simulink model "gm_sampleModel1821_4_sub_sub_sub"  (R2023a)
settings: Solver=VariableStepAuto  StartTime=0.0  StopTime=10.0  RelTol=1e-3
libraries: hdlsllib x3
settings Model: Creator=user1  LastModifiedBy=user1
settings OptimizationCC: BlockReduction=off  ConditionallyExecuteInputs=off
settings DebuggingCC: InheritedTsInSrcMsg=none

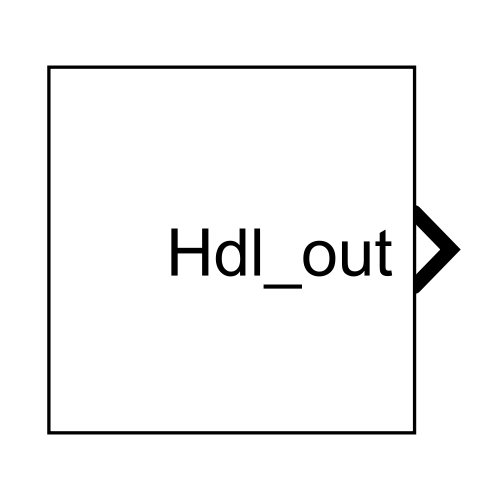
[thumbnail: Simulink's stored preview of the top-level diagram]
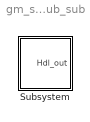
== system gm_sampleModel1821_4_sub_sub_sub ==
  Subsystem : Subsystem

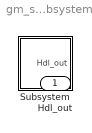
== system gm_sampleModel1821_4_sub_sub_sub/Subsystem ==
  Subsystem : Subsystem
  Hdl_out : Outport  OutDataTypeStr=uint8

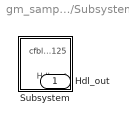
== system gm_sampleModel1821_4_sub_sub_sub/Subsystem/Subsystem ==
  Subsystem : Subsystem
  Hdl_out : Outport  OutDataTypeStr=uint8

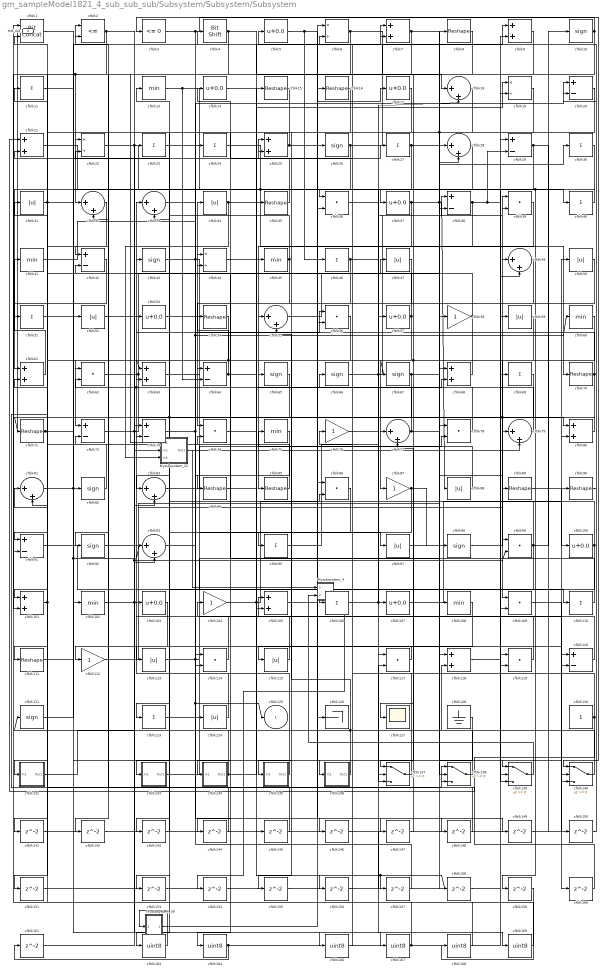
== system gm_sampleModel1821_4_sub_sub_sub/Subsystem/Subsystem/Subsystem ==
  Mysubsystem_22 : Subsystem  TreatAsAtomicUnit=on  RTWFcnName=Mysubsystem_22
      settings: RTWFcnNameOpts=User specified  RTWFileNameOpts=Use function name
  Mysubsystem_39 : Subsystem  TreatAsAtomicUnit=on  RTWFcnName=Mysubsystem_39
      settings: RTWFcnNameOpts=User specified  RTWFileNameOpts=Use function name
  Mysubsystem_4 : Subsystem  TreatAsAtomicUnit=on  RTWFcnName=Mysubsystem_4
      settings: RTWFcnNameOpts=User specified  RTWFileNameOpts=Use function name
  cfblk1 : hdlsllib/Logic and Bit Operations/Bit Concat  numInputs=2
  cfblk{10,26,43,65..67,82,92,98,121} (10 alike) : Signum
  cfblk{5,14,17,37,53,57,100,103,107} (9 alike) : Bias  Bias=0.0  SaturateOnIntegerOverflow=off
  cfblk{7,9,21,25,61,63,68,80,101,105,118} (11 alike) : Sum  OutDataTypeStr=uint8
  cfblk{13,41,45,60,75,102,108} (7 alike) : MinMax  OutDataTypeStr=uint8
  cfblk{58,76,87,104,112} (5 alike) : Gain  OutDataTypeStr=uint8
  cfblk{11,23..24,27,30,40,46,51,69,95,106,110,123} (13 alike) : Sum  Inputs=+  OutDataTypeStr=uint8
  cfblk{36,39,56,62,74,78,86,99,109,114,117,119} (12 alike) : DotProduct  OutDataTypeStr=uint8
  cfblk{8,15..16,35,54,70..71,84..85,89..90,111} (12 alike) : Reshape
  cfblk{31,34,47,50,52,59,88,97,113,115,124} (11 alike) : Abs  OutDataTypeStr=uint8  SaturateOnIntegerOverflow=off
  cfblk{20,29,38,42,64,72..73,91,120} (9 alike) : Sum  Inputs=+-  OutDataTypeStr=uint8
  cfblk126 : Terminator
  cfblk127 : Scope
  cfblk128 : Ground
  cfblk130 : Constant  OutDataTypeStr=uint8  SampleTime=-1
  cfblk131 : Subsystem
      settings: LibrarySourceBlock=|
      | hdlsllib/Ports &
      | Subsystems/Subsystem
  cfblk133 : Subsystem
      settings: LibrarySourceBlock=|
      | hdlsllib/Ports &
      | Subsystems/Subsystem
  cfblk134 : Subsystem
      settings: LibrarySourceBlock=|
      | hdlsllib/Ports &
      | Subsystems/Subsystem
  cfblk135 : Subsystem
      settings: LibrarySourceBlock=|
      | hdlsllib/Ports &
      | Subsystems/Subsystem
  cfblk136 : Subsystem
      settings: LibrarySourceBlock=|
      | hdlsllib/Ports &
      | Subsystems/Subsystem
  cfblk{137..140} (4 alike) : Switch  OutDataTypeStr=uint8  SaturateOnIntegerOverflow=off  InputSameDT=off
  cfblk{141..151,153..161} (20 alike) : Delay  SampleTime=1
  cfblk{163..164,166..169} (6 alike) : DataTypeConversion  OutDataTypeStr=uint8  SaturateOnIntegerOverflow=off  RndMeth=Floor
  cfblk{18,28,32..33,49,55,77,79,81,83,93} (11 alike) : Sum  Inputs=|++  OutDataTypeStr=uint8
  cfblk{6,19,22,44} (4 alike) : Product  Inputs=*/  OutDataTypeStr=uint8  RndMeth=Zero  SaturateOnIntegerOverflow=on
  cfblk2 : RelationalOperator  Operator=<=  OutDataTypeStr=boolean  InputSameDT=off
  cfblk3 : hdlsllib/Logic and Bit Operations/Compare To Zero  relop=<=  OutDataTypeStr=uint8
  cfblk4 : hdlsllib/Logic and Bit Operations/Bit Shift  mode=Shift Left Logical  N=0
  cfblk125 : Outport  OutDataTypeStr=uint8  VectorParamsAs1DForOutWhenUnconnected=off
  Hdl_out : Outport  Port=2  OutDataTypeStr=uint8
  wires:
  Mysubsystem_39/1(Out1) -> cfblk86/1
  cfblk163/1 -> Mysubsystem_39/1(In1)
  Mysubsystem_22/1(Out1) -> Mysubsystem_4/1(In1)
  Mysubsystem_4/1(Out1) -> cfblk154/1
  cfblk139/1 -> Mysubsystem_4/2(In2)
  cfblk169/1 -> cfblk1/2
  cfblk146/1 -> cfblk169/1
  cfblk168/1 -> cfblk1/1
  cfblk159/1 -> cfblk168/1
  cfblk167/1 -> cfblk49/2, cfblk73/1
  cfblk166/1 -> cfblk86/2
  cfblk164/1 -> cfblk161/1, cfblk59/1
  cfblk161/1 -> cfblk93/2
  cfblk160/1 -> cfblk138/3
  cfblk109/1 -> cfblk160/1
  cfblk158/1 -> cfblk19/2
  cfblk157/1 -> cfblk114/1
  cfblk156/1 -> cfblk119/1
  cfblk155/1 -> cfblk56/2
  cfblk154/1 -> cfblk78/1
  cfblk153/1 -> cfblk6/1
  cfblk16/1 -> cfblk153/1
  cfblk151/1 -> cfblk117/2
  cfblk150/1 -> cfblk20/2
  cfblk149/1 -> cfblk80/2
  cfblk148/1 -> cfblk81/1
  cfblk147/1 -> cfblk77/2
  cfblk33/1 -> cfblk147/1
  cfblk145/1 -> cfblk32/2
  cfblk14/1 -> cfblk145/1
  cfblk144/1 -> cfblk72/2
  cfblk108/1 -> cfblk144/1
  cfblk143/1 -> cfblk73/2
  cfblk142/1 -> cfblk83/2
  cfblk15/1 -> cfblk142/1
  cfblk141/1 -> cfblk120/1
  cfblk54/1 -> cfblk141/1
  cfblk110/1 -> cfblk74/2
  cfblk29/1 -> cfblk150/1, cfblk151/1
  cfblk19/1 -> cfblk101/1
  cfblk118/1 -> cfblk9/2
  cfblk69/1 -> cfblk99/1
  cfblk100/1 -> cfblk109/2, cfblk21/2
  cfblk93/1 -> cfblk20/1
  cfblk87/1 -> cfblk133/1(In1), cfblk98/1
  cfblk42/1 -> cfblk91/1
  cfblk4/1 -> Mysubsystem_22/1(In1), cfblk18/1
  cfblk11/1 -> cfblk4/1
  cfblk75/1 -> cfblk114/2
  cfblk84/1 -> cfblk68/2
  cfblk115/1 -> cfblk103/1
  cfblk32/1 -> cfblk111/1
  cfblk28/1 -> cfblk54/1
  cfblk101/1 -> cfblk61/2, cfblk131/1(In1)
  cfblk131/1(Out1) -> cfblk23/1
  cfblk30/1 -> cfblk42/1, cfblk159/1
  cfblk106/1 -> cfblk137/2, cfblk18/2
  cfblk6/1 -> cfblk58/1, cfblk101/2
  cfblk120/1 -> cfblk6/2
  cfblk71/1 -> cfblk136/1(In1), Hdl_out/1
  cfblk22/1 -> Mysubsystem_22/2(In2), cfblk68/1
  cfblk99/1 -> cfblk10/1, cfblk44/1, cfblk143/1
  cfblk21/1 -> cfblk107/1
  cfblk62/1 -> cfblk35/1, cfblk124/1
  cfblk140/1 -> cfblk118/2
  cfblk117/1 -> cfblk113/1
  cfblk73/1 -> cfblk125/1, cfblk139/1, cfblk56/1, cfblk60/1
  cfblk76/1 -> cfblk120/2
  cfblk35/1 -> cfblk14/1
  cfblk77/1 -> cfblk108/1, cfblk42/2
  cfblk105/1 -> cfblk17/1
  cfblk38/1 -> cfblk137/1, cfblk67/1, cfblk29/2, cfblk140/3
  cfblk43/1 -> cfblk126/1, cfblk146/1
  cfblk111/1 -> cfblk102/1
  cfblk9/1 -> cfblk92/1
  cfblk78/1 -> cfblk2/2, cfblk63/2
  cfblk74/1 -> cfblk157/1, cfblk158/1
  cfblk55/1 -> cfblk47/1
  cfblk36/1 -> cfblk57/1
  cfblk56/1 -> cfblk65/1
  cfblk82/1 -> cfblk31/1
  cfblk79/1 -> cfblk2/1
  cfblk49/1 -> cfblk105/2
  cfblk1/1 -> cfblk167/1
  cfblk91/1 -> cfblk106/1
  cfblk65/1 -> cfblk123/1, cfblk81/2
  cfblk51/1 -> cfblk7/1
  cfblk52/1 -> cfblk28/2
  cfblk86/1 -> cfblk164/1
  cfblk89/1 -> cfblk100/1
  cfblk103/1 -> cfblk112/1
  cfblk119/1 -> cfblk66/1
  cfblk85/1 -> cfblk62/2
  cfblk67/1 -> cfblk140/2, cfblk163/1
  cfblk95/1 -> cfblk38/1
  cfblk41/1 -> cfblk24/1
  cfblk92/1 -> cfblk49/1
  cfblk34/1 -> Mysubsystem_22/3(In3), cfblk156/1
  cfblk5/1 -> cfblk46/1, cfblk149/1
  cfblk130/1 -> cfblk21/1, cfblk25/1
  cfblk133/1(Out1) -> cfblk90/1
  cfblk136/1(Out1) -> cfblk121/1, cfblk55/2
  cfblk114/1 -> cfblk104/1
  cfblk10/1 -> cfblk77/1, cfblk3/1
  cfblk57/1 -> cfblk11/1, cfblk155/1
  cfblk97/1 -> cfblk29/1
  cfblk17/1 -> cfblk84/1
  cfblk121/1 -> cfblk52/1, cfblk93/1
  cfblk98/1 -> cfblk39/2
  cfblk66/1 -> cfblk39/1, cfblk139/3
  cfblk83/1 -> cfblk78/2
  cfblk25/1 -> cfblk22/1, cfblk139/2
  cfblk123/1 -> cfblk8/1
  cfblk3/1 -> cfblk140/1, cfblk148/1
  cfblk68/1 -> cfblk62/1
  cfblk138/1 -> cfblk76/1
  cfblk72/1 -> cfblk80/1, cfblk79/2
  cfblk70/1 -> cfblk95/1, cfblk53/1
  cfblk128/1 -> cfblk138/2
  cfblk61/1 -> cfblk41/1
  cfblk26/1 -> cfblk9/1, cfblk134/1(In1)
  cfblk112/1 -> cfblk28/1
  cfblk23/1 -> cfblk37/1
  cfblk102/1 -> cfblk99/2, cfblk44/2, cfblk15/1
  cfblk60/1 -> cfblk109/1
  cfblk31/1 -> cfblk138/1, cfblk40/1
  cfblk137/1 -> cfblk105/1
  cfblk45/1 -> cfblk13/1, cfblk64/1
  cfblk134/1(Out1) -> cfblk33/2, cfblk19/1
  cfblk124/1 -> cfblk43/1
  cfblk20/1 -> cfblk83/1, cfblk38/2
  cfblk113/1 -> cfblk26/1, cfblk27/1
  cfblk39/1 -> cfblk45/1
  cfblk18/1 -> cfblk135/1(In1)
  cfblk46/1 -> cfblk117/1, cfblk115/1
  cfblk80/1 -> cfblk71/1, cfblk79/1
  cfblk50/1 -> cfblk74/1
  cfblk44/1 -> cfblk55/1
  cfblk88/1 -> cfblk75/1
  cfblk7/1 -> cfblk118/1, cfblk91/2
  cfblk27/1 -> cfblk61/1, cfblk89/1
  cfblk8/1 -> cfblk127/1
  cfblk59/1 -> cfblk87/1
  cfblk135/1(Out1) -> cfblk33/1
  cfblk13/1 -> cfblk36/2, cfblk64/2
  cfblk104/1 -> cfblk16/1, cfblk119/2
  cfblk40/1 -> cfblk36/1
  cfblk53/1 -> cfblk97/1
  cfblk64/1 -> cfblk34/1, cfblk63/1, cfblk7/2
  cfblk58/1 -> cfblk72/1, cfblk22/2
  cfblk107/1 -> cfblk50/1
  cfblk90/1 -> cfblk5/1
  cfblk37/1 -> cfblk88/1, cfblk30/1, cfblk137/3
  cfblk63/1 -> cfblk110/1
  cfblk2/1 -> cfblk32/1, cfblk51/1, cfblk166/1
  cfblk81/1 -> cfblk82/1, cfblk25/2
  cfblk24/1 -> cfblk70/1, cfblk69/1
  cfblk47/1 -> cfblk85/1

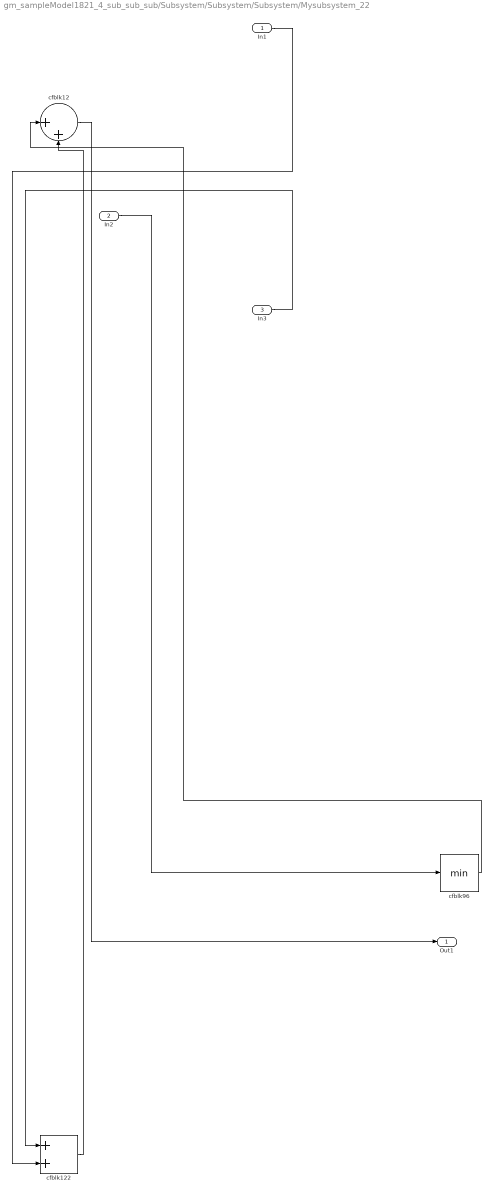
== system gm_sampleModel1821_4_sub_sub_sub/Subsystem/Subsystem/Subsystem/Mysubsystem_22 ==
  In1 : Inport
  In2 : Inport  Port=2
  In3 : Inport  Port=3
  cfblk12 : Sum  Inputs=|++
  cfblk122 : Sum
  cfblk96 : MinMax
  Out1 : Outport
  wires:
  cfblk122/1 -> cfblk12/2
  In3/1 -> cfblk122/1
  cfblk96/1 -> cfblk12/1
  In1/1 -> cfblk122/2
  cfblk12/1 -> Out1/1
  In2/1 -> cfblk96/1

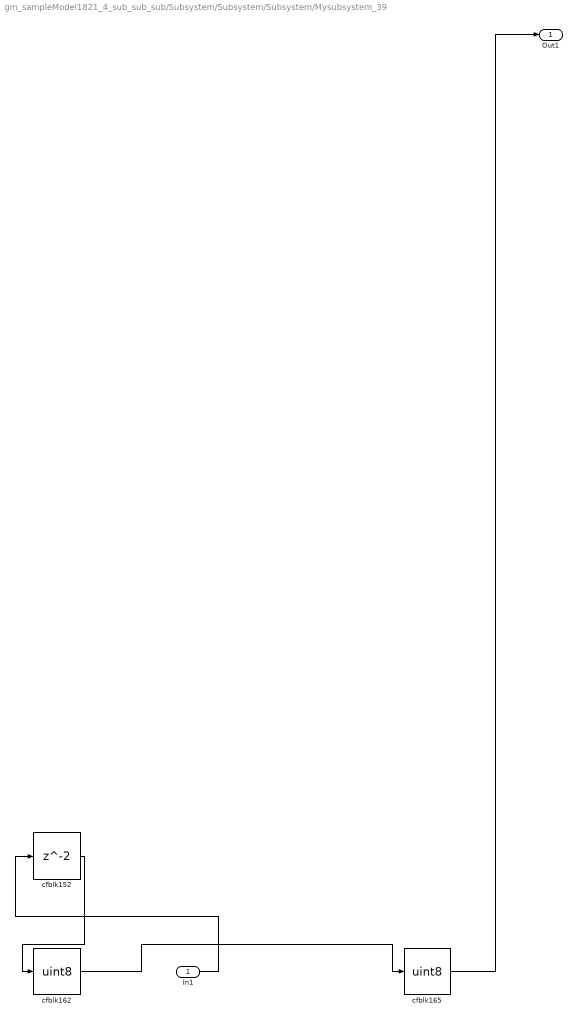
== system gm_sampleModel1821_4_sub_sub_sub/Subsystem/Subsystem/Subsystem/Mysubsystem_39 ==
  In1 : Inport
  cfblk152 : Delay  SampleTime=1
  cfblk162 : DataTypeConversion  OutDataTypeStr=uint8  SaturateOnIntegerOverflow=off  RndMeth=Floor
  cfblk165 : DataTypeConversion  OutDataTypeStr=uint8  SaturateOnIntegerOverflow=off  RndMeth=Floor
  Out1 : Outport
  wires:
  cfblk152/1 -> cfblk162/1
  cfblk162/1 -> cfblk165/1
  cfblk165/1 -> Out1/1
  In1/1 -> cfblk152/1

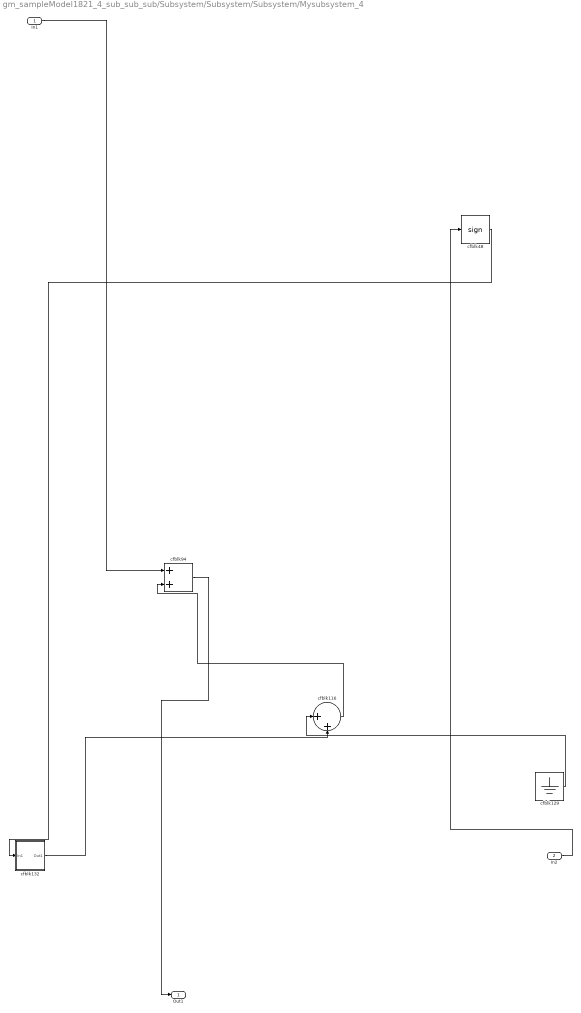
== system gm_sampleModel1821_4_sub_sub_sub/Subsystem/Subsystem/Subsystem/Mysubsystem_4 ==
  In1 : Inport
  In2 : Inport  Port=2
  cfblk116 : Sum  Inputs=|++
  cfblk129 : Ground
  cfblk132 : Subsystem
      settings: LibrarySourceBlock=|
      | hdlsllib/Ports &
      | Subsystems/Subsystem
  cfblk48 : Signum
  cfblk94 : Sum
  Out1 : Outport
  wires:
  cfblk116/1 -> cfblk94/2
  cfblk48/1 -> cfblk132/1(In1)
  cfblk132/1(Out1) -> cfblk116/2
  cfblk129/1 -> cfblk116/1
  In2/1 -> cfblk48/1
  In1/1 -> cfblk94/1
  cfblk94/1 -> Out1/1

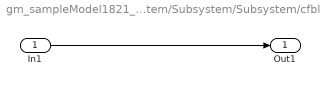
== system gm_sampleModel1821_4_sub_sub_sub/Subsystem/Subsystem/Subsystem/cfblk131 ==
  In1 : Inport
  Out1 : Outport
  wires:
  In1/1 -> Out1/1

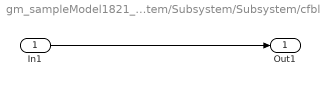
== system gm_sampleModel1821_4_sub_sub_sub/Subsystem/Subsystem/Subsystem/cfblk133 ==
  In1 : Inport
  Out1 : Outport
  wires:
  In1/1 -> Out1/1

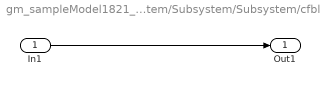
== system gm_sampleModel1821_4_sub_sub_sub/Subsystem/Subsystem/Subsystem/cfblk134 ==
  In1 : Inport
  Out1 : Outport
  wires:
  In1/1 -> Out1/1

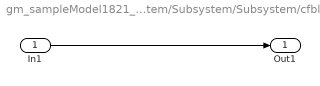
== system gm_sampleModel1821_4_sub_sub_sub/Subsystem/Subsystem/Subsystem/cfblk135 ==
  In1 : Inport
  Out1 : Outport
  wires:
  In1/1 -> Out1/1

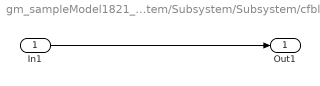
== system gm_sampleModel1821_4_sub_sub_sub/Subsystem/Subsystem/Subsystem/cfblk136 ==
  In1 : Inport
  Out1 : Outport
  wires:
  In1/1 -> Out1/1

== system gm_sampleModel1821_4_sub_sub_sub/Subsystem/Subsystem/Subsystem/Mysubsystem_4/cfblk132 ==
  In1 : Inport
  Out1 : Outport
  wires:
  In1/1 -> Out1/1
